simulink model "Automated_features1"  (R2020b)
settings: Solver=VariableStepAuto  StartTime=0.0  StopTime=10.0  RelTol=1e-3
undefined symbols (not defined in the file): sigbuilder_block
libraries: simulink x126
(part 2 of 3)

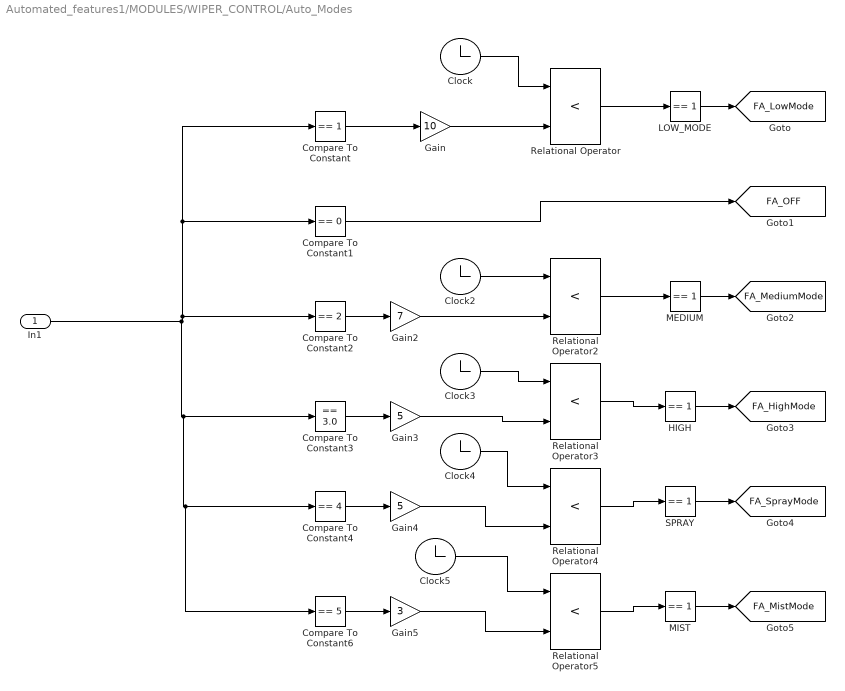
== system Automated_features1/MODULES/WIPER_CONTROL/Auto_Modes ==
  In1 : Inport
  Clock{,2..5} (5 alike) : Clock
      settings: Decimation=5
  Compare To Constant : simulink/Logic and Bit Operations/Compare To Constant  relop===  const=1  OutDataTypeStr=boolean
  Compare To Constant1 : simulink/Logic and Bit Operations/Compare To Constant  relop===  const=0  OutDataTypeStr=boolean
  Compare To Constant2 : simulink/Logic and Bit Operations/Compare To Constant  relop===  const=2  OutDataTypeStr=boolean
  Compare To Constant3 : simulink/Logic and Bit Operations/Compare To Constant  relop===  const=3.0  OutDataTypeStr=boolean
  Compare To Constant4 : simulink/Logic and Bit Operations/Compare To Constant  relop===  const=4  OutDataTypeStr=boolean
  Compare To Constant6 : simulink/Logic and Bit Operations/Compare To Constant  relop===  const=5  OutDataTypeStr=boolean
  Gain : Gain  Gain=10
  Gain2 : Gain  Gain=7
  Gain3 : Gain  Gain=5
  Gain4 : Gain  Gain=5
  Gain5 : Gain  Gain=3
  HIGH : simulink/Logic and Bit Operations/Compare To Constant  relop===  const=1  OutDataTypeStr=boolean
  LOW_MODE : simulink/Logic and Bit Operations/Compare To Constant  relop===  const=1  OutDataTypeStr=boolean
  MEDIUM : simulink/Logic and Bit Operations/Compare To Constant  relop===  const=1  OutDataTypeStr=boolean
  MIST : simulink/Logic and Bit Operations/Compare To Constant  relop===  const=1  OutDataTypeStr=boolean
  Relational Operator{,2..5} (5 alike) : RelationalOperator  Operator=<  OutDataTypeStr=boolean  RndMeth=Simplest
  SPRAY : simulink/Logic and Bit Operations/Compare To Constant  relop===  const=1  OutDataTypeStr=boolean
  tag scope: FA_HighMode=global, FA_LowMode=global, FA_MediumMode=global, FA_MistMode=global, FA_OFF=global, FA_SprayMode=global
  wires:
  In1/1 -> Compare To Constant6/1, Compare To Constant4/1, Compare To Constant3/1, Compare To Constant2/1, Compare To Constant/1, Compare To Constant1/1
  Clock/1 -> Relational Operator/1
  Relational Operator/1 -> LOW_MODE/1
  Gain/1 -> Relational Operator/2
  Compare To Constant/1 -> Gain/1
  Clock2/1 -> Relational Operator2/1
  Gain2/1 -> Relational Operator2/2
  Compare To Constant2/1 -> Gain2/1
  Clock3/1 -> Relational Operator3/1
  Gain3/1 -> Relational Operator3/2
  Compare To Constant3/1 -> Gain3/1
  Gain4/1 -> Relational Operator4/2
  Clock4/1 -> Relational Operator4/1
  Compare To Constant4/1 -> Gain4/1
  LOW_MODE/1 -> [FA_LowMode]
  MEDIUM/1 -> [FA_MediumMode]
  Relational Operator2/1 -> MEDIUM/1
  HIGH/1 -> [FA_HighMode]
  Relational Operator3/1 -> HIGH/1
  SPRAY/1 -> [FA_SprayMode]
  Relational Operator4/1 -> SPRAY/1
  Compare To Constant1/1 -> [FA_OFF]
  Relational Operator5/1 -> MIST/1
  Gain5/1 -> Relational Operator5/2
  Clock5/1 -> Relational Operator5/1
  MIST/1 -> [FA_MistMode]
  Compare To Constant6/1 -> Gain5/1

== system Automated_features1/MODULES/WIPER_CONTROL/Back_Windshield ==
  Lamp : LampBlock

== system Automated_features1/MODULES/WIPER_CONTROL/Front_Windshield ==
  Enable : EnablePort
  Auto_Modes : Subsystem
  Manual_mode : Subsystem
  Rotary Switch : RotarySwitchBlock  Commented=on
      settings: Values={{'Off', 'Low', 'Medium', 'High', 'Spray', 'Manual', 'MistMode'}, [0 1 2 3 4 5 6]}
  wires:
  [FW_Modes] -> Manual_mode/1(In1), Auto_Modes/1(In1)

== system Automated_features1/MODULES/WIPER_CONTROL/Manual_mode ==
  In1 : Inport
  Bw30_60 : Logic  IconShape=distinctive  AllPortsSameDT=off  OutDataTypeStr=boolean
  Bw60_100 : Logic  IconShape=distinctive  AllPortsSameDT=off  OutDataTypeStr=boolean
  Compare To Constant1 : simulink/Logic and Bit Operations/Compare To Constant  relop=>  const=30  OutDataTypeStr=boolean
  Compare To Constant2 : simulink/Logic and Bit Operations/Compare To Constant  relop=<=  const=60  OutDataTypeStr=boolean
  Compare To Constant3 : simulink/Logic and Bit Operations/Compare To Constant  relop=>  const=60  OutDataTypeStr=boolean
  Compare To Constant4 : simulink/Logic and Bit Operations/Compare To Constant  relop=<=  const=100  OutDataTypeStr=boolean
  Display : Display
  LessThan30 : simulink/Logic and Bit Operations/Compare To Constant  relop=<=  const=30  OutDataTypeStr=boolean
  Slider : SliderBlock
  String Constant : StringConstant  String="\"Undefined!\""
  Switch : Switch  Criteria=u2 > Threshold  Threshold=5
  tag scope: FM_Bw30_60=global, FM_Bw60_100=global, FM_lessthan30=global
  wires:
  Compare To Constant1/1 -> Bw30_60/1
  Bw30_60/1 -> [FM_Bw30_60]
  [FC_ManualInput] -> Compare To Constant4/1, Compare To Constant3/1, Compare To Constant2/1, Compare To Constant1/1, LessThan30/1, Switch/1
  Compare To Constant4/1 -> Bw60_100/2
  LessThan30/1 -> [FM_lessthan30]
  Switch/1 -> Display/1
  Compare To Constant3/1 -> Bw60_100/1
  Bw60_100/1 -> [FM_Bw60_100]
  Compare To Constant2/1 -> Bw30_60/2
  In1/1 -> Switch/2
  String Constant/1 -> Switch/3

== system Automated_features1/MODULES/WIPER_CONTROL/Wiper_Control ==
  Inport : Inport
  AND : Logic  IconShape=distinctive  AllPortsSameDT=off  OutDataTypeStr=boolean
  AND1 : Logic  IconShape=distinctive  AllPortsSameDT=off  OutDataTypeStr=boolean
  Atomic Subsystem : Subsystem  TreatAsAtomicUnit=on
  Atomic Subsystem1 : Subsystem  TreatAsAtomicUnit=on
  Back switch : SliderSwitchBlock  Commented=on
      settings: Values={{'Off', 'On'}, [0 1]}
  Back_Windshield : Subsystem  Commented=on  TreatAsAtomicUnit=on
  Front switch : SliderSwitchBlock  Commented=on
      settings: Values={{'Off', 'On'}, [0 1]}
  Front_Windshield : Subsystem  Commented=on  TreatAsAtomicUnit=on
  wires:
  Inport/1 -> AND1/2, AND/2
  [WC_FrontS] -> AND/1
  [WC_BackS] -> AND1/1
  AND1/1 -> Atomic Subsystem/1(Inport)
  AND/1 -> Atomic Subsystem1/1(Inport)

== system Automated_features1/MODULES/sunroof/Subsystem ==
  Enable : Inport
  Inport : Inport  Port=2
  Enabled Subsystem : Subsystem  TreatAsAtomicUnit=on
  Outport : Outport
  wires:
  Enabled Subsystem/1(Outport) -> Outport/1
  Inport/1 -> Enabled Subsystem/1(In1)
  Enable/1 -> Enabled Subsystem/Enable

== system Automated_features1/MODULES/sunroof/Subsystem1 ==
  Enable : Inport
  Inport : Inport  Port=2
  Enabled Subsystem1 : Subsystem  TreatAsAtomicUnit=on
  Outport : Outport
  wires:
  Inport/1 -> Enabled Subsystem1/1(In1)
  Enabled Subsystem1/1(Outport) -> Outport/1
  Enable/1 -> Enabled Subsystem1/Enable

== system Automated_features1/MODULES/sunroof/enabling system ==
  Chart : Stateflow chart  TreatAsAtomicUnit=on
      settings: PortSchema="{\"entries\":[{\"content\":{\"sides\":[{\"content\":{\"connectorIds\":[\"In2\",\"In1\"]},\"type\":\"ConnectorPlacement.EquallySpacedRectSide\",\"uuid\":\"e77fb548-5411-4dff-a09c-dcff2e4e83fa\"},{\"content\":{\"connectorIds\":[\"Out1\",\"Out2\"],\"side\":\"RIGHT\"},\"type\":\"ConnectorPlacement.EquallySpacedRectSide\",\"uuid\":\"fb2d12f5-730f-4265-a3f8-30409b75040e\"},{\"content\":{\"connectorIds\":[],\"side\":\"TOP\"},\"type\":\"ConnectorPlacement.EquallySpacedRectSide\",\"uuid\":\"5ec706c6-4a0b-4294-a183-09121d2d4adc\"},{\"content\":{\"connectorIds\":[],\"side\":\"HIDDEN\"},\"type\":\"ConnectorPlacement.EquallySpacedRectSide\",\"uuid\":\"e64ccab7-f9d3-41b0-81fa-c7461dca4746\"}]},\"type\":\"ConnectorPlacement.EquallySpacedConnector\",\"uuid\":\"e8c87857-404b-4a97-9417-fff31936aad1\"}],\"packageUris\":[\"http://schema.mathworks.com/mf0/Connector/R2020b\"],\"version\":\"1.0\"}"
  Outport : Outport
  enableO : Outport  Port=2
  wires:
  Chart/1(enableC) -> Outport/1
  [CL_SW] -> Chart/1(closeButton)
  Chart/2(enableO) -> enableO/1
  [OP_SW] -> Chart/2(openButton)

== system Automated_features1/MODULES/	POWER_WINDOW/Subsystem4/Front_left_subsystem ==
  lock/unlock : Inport
  In_fl_b : Inport  Port=2
  In_fl_Dc : Inport  Port=3
  object : Inport  Port=4
  Enable : EnablePort
  AND : Logic  IconShape=distinctive  AllPortsSameDT=off  OutDataTypeStr=boolean
  Compare To Constant1 : simulink/Logic and Bit Operations/Compare To Constant  relop===  const=1  OutDataTypeStr=boolean
  Display : Display
  Display1 : Display
  Scope : Scope  NumInputPorts=2
  Switch_lock_unlock : Switch  Criteria=u2 > Threshold
  check_ip : Constant
  decision_Box : Stateflow chart  TreatAsAtomicUnit=on
  inp_data : Logic  Operator=NXOR  IconShape=distinctive  AllPortsSameDT=off  OutDataTypeStr=boolean
  or1 : Logic  Operator=NXOR  IconShape=distinctive  AllPortsSameDT=off  OutDataTypeStr=boolean
  Outport : Outport
  Outport1 : Outport  Port=2
  tag scope: A=global
  wires:
  In_fl_b/1 -> AND/1
  check_ip/1 -> or1/1
  Switch_lock_unlock/1 -> [b1]
  Compare To Constant1/1 -> or1/2
  [b1] -> Display/1
  decision_Box/1(op1) -> Outport1/1, Switch_lock_unlock/3, Switch_lock_unlock/1, Scope/2, [A]
  decision_Box/2(warning) -> Outport/1, Scope/1
  object/1 -> decision_Box/2(data1)
  [A] -> Display1/1
  inp_data/1 -> decision_Box/1(data)
  In_fl_Dc/1 -> Compare To Constant1/1
  AND/1 -> inp_data/1  "res"
  or1/1 -> inp_data/2
  lock/unlock/1 -> Switch_lock_unlock/2, AND/2

== system Automated_features1/MODULES/	POWER_WINDOW/Subsystem4/Rear_right_Subsystem ==
  lock/unlock : Inport
  In2 : Inport  Port=2
  In3 : Inport  Port=3
  object : Inport  Port=4
  Enable : EnablePort
  Chart : Stateflow chart  TreatAsAtomicUnit=on
  Compare To Constant1 : simulink/Logic and Bit Operations/Compare To Constant  relop===  const=3  OutDataTypeStr=boolean
  Constant1 : Constant  Value=3
  Display2 : Display
  Display3 : Display
  Scope : Scope  NumInputPorts=2
  Switch : Switch  Criteria=u2 > Threshold
  or1 : Logic  Operator=NXOR  IconShape=distinctive  AllPortsSameDT=off  OutDataTypeStr=boolean
  or2 : Logic  IconShape=distinctive  AllPortsSameDT=off  OutDataTypeStr=boolean
  or3 : Logic  Operator=NXOR  IconShape=distinctive  AllPortsSameDT=off  OutDataTypeStr=boolean
  Outport : Outport
  Outport1 : Outport  Port=2
  tag scope: c=global
  wires:
  Constant1/1 -> or1/1
  [b3] -> Display2/1
  Compare To Constant1/1 -> or1/2
  Switch/1 -> [b3]
  lock/unlock/1 -> or2/2, Switch/2
  Chart/2(warning) -> Scope/1, Outport/1  "ss3"
  object/1 -> Chart/2(data1)
  or1/1 -> or3/2
  or2/1 -> or3/1  "res"
  or3/1 -> Chart/1(data)
  [c] -> Display3/1
  Chart/1(op1) -> Outport1/1, [c], Scope/2, Switch/3, Switch/1
  In2/1 -> or2/1
  In3/1 -> Compare To Constant1/1

== system Automated_features1/MODULES/	POWER_WINDOW/Subsystem4/driver_control_Subsystem ==
  In1 : Inport
  object : Inport  Port=2
  Enable : EnablePort
  Chart : Stateflow chart  TreatAsAtomicUnit=on
  Display4 : Display
  Scope : Scope  NumInputPorts=2
  Outport : Outport
  Outport1 : Outport  Port=2
  tag scope: d=global
  wires:
  Chart/2(warning) -> Outport/1, Scope/1  "ss4"
  object/1 -> Chart/2(data1)
  In1/1 -> Chart/1(data)
  [d] -> Display4/1
  Chart/1(op1) -> Outport1/1, [d], Scope/2

== system Automated_features1/MODULES/	POWER_WINDOW/Subsystem4/rear_left_Subsystem ==
  lock/unlock : Inport
  In2 : Inport  Port=2
  In3 : Inport  Port=3
  object : Inport  Port=4
  Enable : EnablePort
  Chart : Stateflow chart  TreatAsAtomicUnit=on
  Compare To Constant2 : simulink/Logic and Bit Operations/Compare To Constant  relop===  const=2  OutDataTypeStr=boolean
  Constant1 : Constant  Value=2
  Display1 : Display
  Display2 : Display
  Scope : Scope  NumInputPorts=2
  Switch1 : Switch  Criteria=u2 > Threshold
  or1 : Logic  Operator=NXOR  IconShape=distinctive  AllPortsSameDT=off  OutDataTypeStr=boolean
  or2 : Logic  Operator=NXOR  IconShape=distinctive  AllPortsSameDT=off  OutDataTypeStr=boolean
  or3 : Logic  IconShape=distinctive  AllPortsSameDT=off  OutDataTypeStr=boolean
  Outport : Outport
  Outport1 : Outport  Port=2
  tag scope: b=global
  wires:
  [b2] -> Display1/1
  Constant1/1 -> or2/1
  Compare To Constant2/1 -> or2/2
  Switch1/1 -> [b2]
  lock/unlock/1 -> Switch1/2, or3/2
  object/1 -> Chart/2(data1)
  Chart/2(warning) -> Outport/1, Scope/1  "ss2"
  or3/1 -> or1/1  "res"
  or2/1 -> or1/2
  or1/1 -> Chart/1(data)
  [b] -> Display2/1
  Chart/1(op1) -> Outport1/1, [b], Switch1/3, Switch1/1, Scope/2
  In2/1 -> or3/1
  In3/1 -> Compare To Constant2/1

== system Automated_features1/MODULES/Tire Pressure Monitoring System/TP_Monitoring/indicateHigh1 ==
  Enable : EnablePort
  Constant : Constant  Value=0
  Out1 : Outport
  wires:
  Constant/1 -> Out1/1

== system Automated_features1/MODULES/Tire Pressure Monitoring System/TP_Monitoring/indicateHigh2 ==
  Enable : EnablePort
  Constant : Constant  Value=0
  Out1 : Outport
  wires:
  Constant/1 -> Out1/1

== system Automated_features1/MODULES/Tire Pressure Monitoring System/TP_Monitoring/indicateHigh3 ==
  Enable : EnablePort
  Constant : Constant  Value=0
  Out1 : Outport
  wires:
  Constant/1 -> Out1/1

== system Automated_features1/MODULES/Tire Pressure Monitoring System/TP_Monitoring/indicateHigh4 ==
  Enable : EnablePort
  Constant : Constant  Value=0
  Out1 : Outport
  wires:
  Constant/1 -> Out1/1

== system Automated_features1/MODULES/Tire Pressure Monitoring System/TP_Monitoring/indicateLow1 ==
  Enable : EnablePort
  Constant : Constant
  Out1 : Outport
  wires:
  Constant/1 -> Out1/1

== system Automated_features1/MODULES/Tire Pressure Monitoring System/TP_Monitoring/indicateLow2 ==
  Enable : EnablePort
  Constant : Constant
  Out1 : Outport
  wires:
  Constant/1 -> Out1/1

== system Automated_features1/MODULES/Tire Pressure Monitoring System/TP_Monitoring/indicateLow3 ==
  Enable : EnablePort
  Constant : Constant
  Out1 : Outport
  wires:
  Constant/1 -> Out1/1

== system Automated_features1/MODULES/Tire Pressure Monitoring System/TP_Monitoring/indicateLow4 ==
  Enable : EnablePort
  Constant : Constant
  Out1 : Outport
  wires:
  Constant/1 -> Out1/1

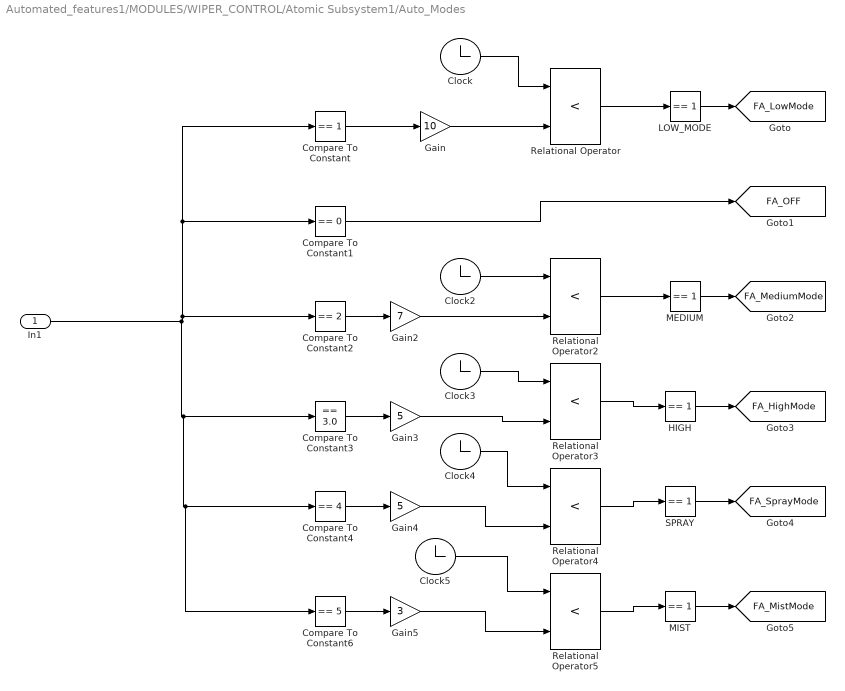
== system Automated_features1/MODULES/WIPER_CONTROL/Atomic Subsystem1/Auto_Modes ==
  In1 : Inport
  Clock{,2..5} (5 alike) : Clock
      settings: Decimation=5
  Compare To Constant : simulink/Logic and Bit Operations/Compare To Constant  relop===  const=1  OutDataTypeStr=boolean
  Compare To Constant1 : simulink/Logic and Bit Operations/Compare To Constant  relop===  const=0  OutDataTypeStr=boolean
  Compare To Constant2 : simulink/Logic and Bit Operations/Compare To Constant  relop===  const=2  OutDataTypeStr=boolean
  Compare To Constant3 : simulink/Logic and Bit Operations/Compare To Constant  relop===  const=3.0  OutDataTypeStr=boolean
  Compare To Constant4 : simulink/Logic and Bit Operations/Compare To Constant  relop===  const=4  OutDataTypeStr=boolean
  Compare To Constant6 : simulink/Logic and Bit Operations/Compare To Constant  relop===  const=5  OutDataTypeStr=boolean
  Gain : Gain  Gain=10
  Gain2 : Gain  Gain=7
  Gain3 : Gain  Gain=5
  Gain4 : Gain  Gain=5
  Gain5 : Gain  Gain=3
  HIGH : simulink/Logic and Bit Operations/Compare To Constant  relop===  const=1  OutDataTypeStr=boolean
  LOW_MODE : simulink/Logic and Bit Operations/Compare To Constant  relop===  const=1  OutDataTypeStr=boolean
  MEDIUM : simulink/Logic and Bit Operations/Compare To Constant  relop===  const=1  OutDataTypeStr=boolean
  MIST : simulink/Logic and Bit Operations/Compare To Constant  relop===  const=1  OutDataTypeStr=boolean
  Relational Operator{,2..5} (5 alike) : RelationalOperator  Operator=<  OutDataTypeStr=boolean  RndMeth=Simplest
  SPRAY : simulink/Logic and Bit Operations/Compare To Constant  relop===  const=1  OutDataTypeStr=boolean
  tag scope: FA_HighMode=global, FA_LowMode=global, FA_MediumMode=global, FA_MistMode=global, FA_OFF=global, FA_SprayMode=global
  wires:
  In1/1 -> Compare To Constant6/1, Compare To Constant4/1, Compare To Constant3/1, Compare To Constant2/1, Compare To Constant/1, Compare To Constant1/1
  Clock/1 -> Relational Operator/1
  Relational Operator/1 -> LOW_MODE/1
  Gain/1 -> Relational Operator/2
  Compare To Constant/1 -> Gain/1
  Clock2/1 -> Relational Operator2/1
  Gain2/1 -> Relational Operator2/2
  Compare To Constant2/1 -> Gain2/1
  Clock3/1 -> Relational Operator3/1
  Gain3/1 -> Relational Operator3/2
  Compare To Constant3/1 -> Gain3/1
  Gain4/1 -> Relational Operator4/2
  Clock4/1 -> Relational Operator4/1
  Compare To Constant4/1 -> Gain4/1
  LOW_MODE/1 -> [FA_LowMode]
  MEDIUM/1 -> [FA_MediumMode]
  Relational Operator2/1 -> MEDIUM/1
  HIGH/1 -> [FA_HighMode]
  Relational Operator3/1 -> HIGH/1
  SPRAY/1 -> [FA_SprayMode]
  Relational Operator4/1 -> SPRAY/1
  Compare To Constant1/1 -> [FA_OFF]
  Relational Operator5/1 -> MIST/1
  Gain5/1 -> Relational Operator5/2
  Clock5/1 -> Relational Operator5/1
  MIST/1 -> [FA_MistMode]
  Compare To Constant6/1 -> Gain5/1

== system Automated_features1/MODULES/WIPER_CONTROL/Atomic Subsystem1/Manual_mode ==
  In1 : Inport
  Bw30_60 : Logic  IconShape=distinctive  AllPortsSameDT=off  OutDataTypeStr=boolean
  Bw60_100 : Logic  IconShape=distinctive  AllPortsSameDT=off  OutDataTypeStr=boolean
  Compare To Constant1 : simulink/Logic and Bit Operations/Compare To Constant  relop=>  const=30  OutDataTypeStr=boolean
  Compare To Constant2 : simulink/Logic and Bit Operations/Compare To Constant  relop=<=  const=60  OutDataTypeStr=boolean
  Compare To Constant3 : simulink/Logic and Bit Operations/Compare To Constant  relop=>  const=60  OutDataTypeStr=boolean
  Compare To Constant4 : simulink/Logic and Bit Operations/Compare To Constant  relop=<=  const=100  OutDataTypeStr=boolean
  Display : Display
  LessThan30 : simulink/Logic and Bit Operations/Compare To Constant  relop=<=  const=30  OutDataTypeStr=boolean
  Slider : SliderBlock
  String Constant : StringConstant  String="\"Undefined!\""
  Switch : Switch  Criteria=u2 > Threshold  Threshold=5
  tag scope: FM_Bw30_60=global, FM_Bw60_100=global, FM_lessthan30=global
  wires:
  Compare To Constant1/1 -> Bw30_60/1
  Bw30_60/1 -> [FM_Bw30_60]
  [FC_ManualInput] -> Compare To Constant4/1, Compare To Constant3/1, Compare To Constant2/1, Compare To Constant1/1, LessThan30/1, Switch/1
  Compare To Constant4/1 -> Bw60_100/2
  LessThan30/1 -> [FM_lessthan30]
  Switch/1 -> Display/1
  Compare To Constant3/1 -> Bw60_100/1
  Bw60_100/1 -> [FM_Bw60_100]
  Compare To Constant2/1 -> Bw30_60/2
  In1/1 -> Switch/2
  String Constant/1 -> Switch/3

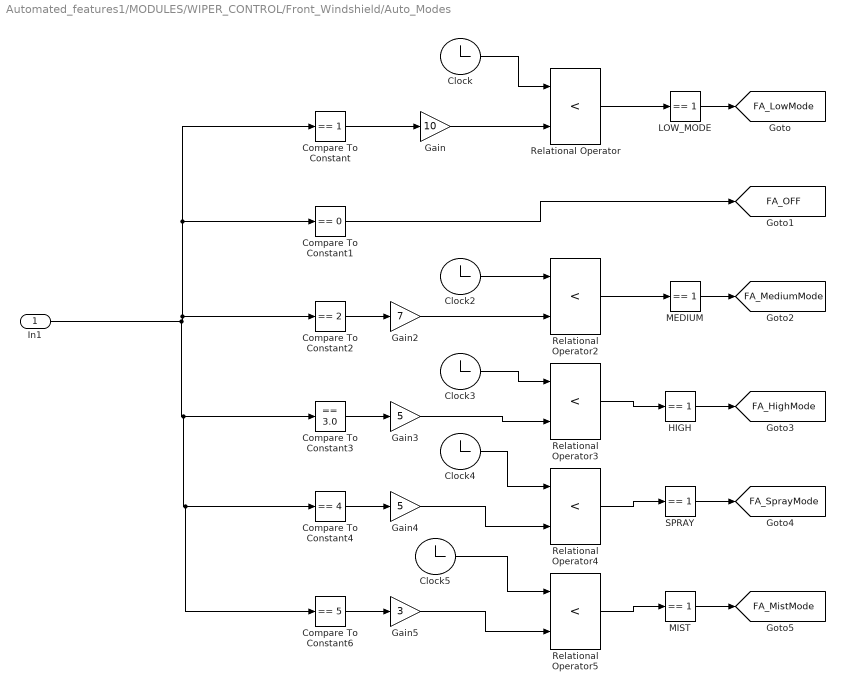
== system Automated_features1/MODULES/WIPER_CONTROL/Front_Windshield/Auto_Modes ==
  In1 : Inport
  Clock{,2..5} (5 alike) : Clock
      settings: Decimation=5
  Compare To Constant : simulink/Logic and Bit Operations/Compare To Constant  relop===  const=1  OutDataTypeStr=boolean
  Compare To Constant1 : simulink/Logic and Bit Operations/Compare To Constant  relop===  const=0  OutDataTypeStr=boolean
  Compare To Constant2 : simulink/Logic and Bit Operations/Compare To Constant  relop===  const=2  OutDataTypeStr=boolean
  Compare To Constant3 : simulink/Logic and Bit Operations/Compare To Constant  relop===  const=3.0  OutDataTypeStr=boolean
  Compare To Constant4 : simulink/Logic and Bit Operations/Compare To Constant  relop===  const=4  OutDataTypeStr=boolean
  Compare To Constant6 : simulink/Logic and Bit Operations/Compare To Constant  relop===  const=5  OutDataTypeStr=boolean
  Gain : Gain  Gain=10
  Gain2 : Gain  Gain=7
  Gain3 : Gain  Gain=5
  Gain4 : Gain  Gain=5
  Gain5 : Gain  Gain=3
  HIGH : simulink/Logic and Bit Operations/Compare To Constant  relop===  const=1  OutDataTypeStr=boolean
  LOW_MODE : simulink/Logic and Bit Operations/Compare To Constant  relop===  const=1  OutDataTypeStr=boolean
  MEDIUM : simulink/Logic and Bit Operations/Compare To Constant  relop===  const=1  OutDataTypeStr=boolean
  MIST : simulink/Logic and Bit Operations/Compare To Constant  relop===  const=1  OutDataTypeStr=boolean
  Relational Operator{,2..5} (5 alike) : RelationalOperator  Operator=<  OutDataTypeStr=boolean  RndMeth=Simplest
  SPRAY : simulink/Logic and Bit Operations/Compare To Constant  relop===  const=1  OutDataTypeStr=boolean
  tag scope: FA_HighMode=global, FA_LowMode=global, FA_MediumMode=global, FA_MistMode=global, FA_OFF=global, FA_SprayMode=global
  wires:
  In1/1 -> Compare To Constant6/1, Compare To Constant4/1, Compare To Constant3/1, Compare To Constant2/1, Compare To Constant/1, Compare To Constant1/1
  Clock/1 -> Relational Operator/1
  Relational Operator/1 -> LOW_MODE/1
  Gain/1 -> Relational Operator/2
  Compare To Constant/1 -> Gain/1
  Clock2/1 -> Relational Operator2/1
  Gain2/1 -> Relational Operator2/2
  Compare To Constant2/1 -> Gain2/1
  Clock3/1 -> Relational Operator3/1
  Gain3/1 -> Relational Operator3/2
  Compare To Constant3/1 -> Gain3/1
  Gain4/1 -> Relational Operator4/2
  Clock4/1 -> Relational Operator4/1
  Compare To Constant4/1 -> Gain4/1
  LOW_MODE/1 -> [FA_LowMode]
  MEDIUM/1 -> [FA_MediumMode]
  Relational Operator2/1 -> MEDIUM/1
  HIGH/1 -> [FA_HighMode]
  Relational Operator3/1 -> HIGH/1
  SPRAY/1 -> [FA_SprayMode]
  Relational Operator4/1 -> SPRAY/1
  Compare To Constant1/1 -> [FA_OFF]
  Relational Operator5/1 -> MIST/1
  Gain5/1 -> Relational Operator5/2
  Clock5/1 -> Relational Operator5/1
  MIST/1 -> [FA_MistMode]
  Compare To Constant6/1 -> Gain5/1

== system Automated_features1/MODULES/WIPER_CONTROL/Front_Windshield/Manual_mode ==
  In1 : Inport
  Bw30_60 : Logic  IconShape=distinctive  AllPortsSameDT=off  OutDataTypeStr=boolean
  Bw60_100 : Logic  IconShape=distinctive  AllPortsSameDT=off  OutDataTypeStr=boolean
  Compare To Constant1 : simulink/Logic and Bit Operations/Compare To Constant  relop=>  const=30  OutDataTypeStr=boolean
  Compare To Constant2 : simulink/Logic and Bit Operations/Compare To Constant  relop=<=  const=60  OutDataTypeStr=boolean
  Compare To Constant3 : simulink/Logic and Bit Operations/Compare To Constant  relop=>  const=60  OutDataTypeStr=boolean
  Compare To Constant4 : simulink/Logic and Bit Operations/Compare To Constant  relop=<=  const=100  OutDataTypeStr=boolean
  Display : Display
  LessThan30 : simulink/Logic and Bit Operations/Compare To Constant  relop=<=  const=30  OutDataTypeStr=boolean
  Slider : SliderBlock
  String Constant : StringConstant  String="\"Undefined!\""
  Switch : Switch  Criteria=u2 > Threshold  Threshold=5
  tag scope: FM_Bw30_60=global, FM_Bw60_100=global, FM_lessthan30=global
  wires:
  Compare To Constant1/1 -> Bw30_60/1
  Bw30_60/1 -> [FM_Bw30_60]
  [FC_ManualInput] -> Compare To Constant4/1, Compare To Constant3/1, Compare To Constant2/1, Compare To Constant1/1, LessThan30/1, Switch/1
  Compare To Constant4/1 -> Bw60_100/2
  LessThan30/1 -> [FM_lessthan30]
  Switch/1 -> Display/1
  Compare To Constant3/1 -> Bw60_100/1
  Bw60_100/1 -> [FM_Bw60_100]
  Compare To Constant2/1 -> Bw30_60/2
  In1/1 -> Switch/2
  String Constant/1 -> Switch/3

== system Automated_features1/MODULES/WIPER_CONTROL/Wiper_Control/Atomic Subsystem ==
  Inport : Inport
  Clock : Clock
      settings: Decimation=5
  Compare To Constant : simulink/Logic and Bit Operations/Compare To Constant  relop===  const=1  OutDataTypeStr=boolean
  Compare To Constant5 : simulink/Logic and Bit Operations/Compare To Constant  relop===  const=1  OutDataTypeStr=boolean
  Gain : Gain  Gain=10
  Relational Operator : RelationalOperator  Operator=<  OutDataTypeStr=boolean  RndMeth=Simplest
  tag scope: BW_Display=global
  wires:
  Compare To Constant5/1 -> [BW_Display]
  Inport/1 -> Compare To Constant/1
  Gain/1 -> Relational Operator/2
  Clock/1 -> Relational Operator/1
  Relational Operator/1 -> Compare To Constant5/1
  Compare To Constant/1 -> Gain/1

== system Automated_features1/MODULES/WIPER_CONTROL/Wiper_Control/Atomic Subsystem1 ==
  Inport : Inport
  Auto_Modes : Subsystem
  Display : Display
  Manual_mode : Subsystem
  wires:
  [FW_Modes] -> Manual_mode/1(In1), Auto_Modes/1(In1)
  Inport/1 -> Display/1

== system Automated_features1/MODULES/WIPER_CONTROL/Wiper_Control/Back_Windshield ==
  Lamp : LampBlock

== system Automated_features1/MODULES/WIPER_CONTROL/Wiper_Control/Front_Windshield ==
  Enable : EnablePort
  Auto_Modes : Subsystem
  Manual_mode : Subsystem
  Rotary Switch : RotarySwitchBlock  Commented=on
      settings: Values={{'Off', 'Low', 'Medium', 'High', 'Spray', 'Manual', 'MistMode'}, [0 1 2 3 4 5 6]}
  wires:
  [FW_Modes] -> Manual_mode/1(In1), Auto_Modes/1(In1)

== system Automated_features1/MODULES/sunroof/Subsystem/Enabled Subsystem ==
  In1 : Inport
  Enable : EnablePort
  Outport : Outport
  wires:
  In1/1 -> Outport/1

== system Automated_features1/MODULES/sunroof/Subsystem1/Enabled Subsystem1 ==
  In1 : Inport
  Enable : EnablePort
  Outport : Outport
  wires:
  In1/1 -> Outport/1

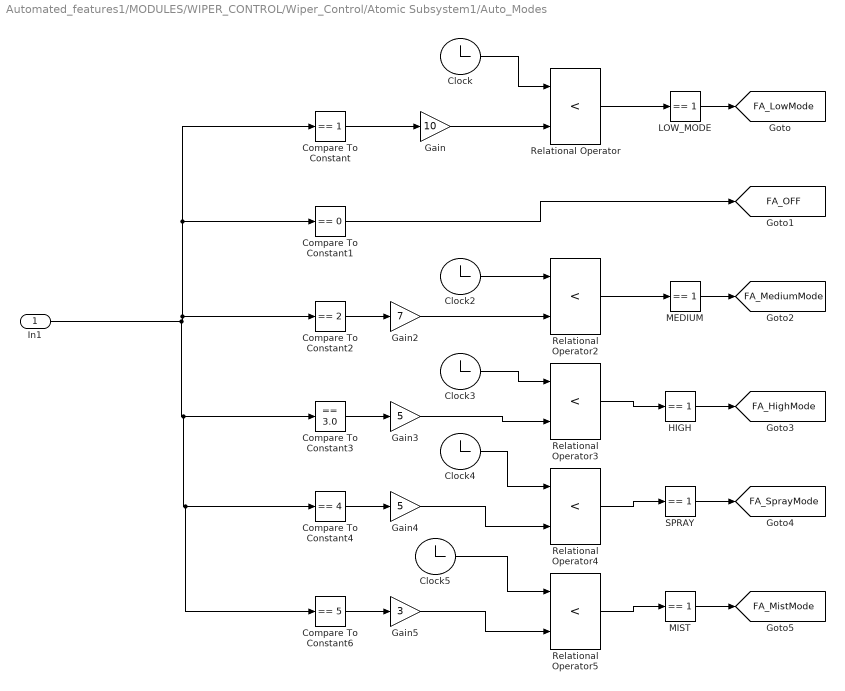
== system Automated_features1/MODULES/WIPER_CONTROL/Wiper_Control/Atomic Subsystem1/Auto_Modes ==
  In1 : Inport
  Clock{,2..5} (5 alike) : Clock
      settings: Decimation=5
  Compare To Constant : simulink/Logic and Bit Operations/Compare To Constant  relop===  const=1  OutDataTypeStr=boolean
  Compare To Constant1 : simulink/Logic and Bit Operations/Compare To Constant  relop===  const=0  OutDataTypeStr=boolean
  Compare To Constant2 : simulink/Logic and Bit Operations/Compare To Constant  relop===  const=2  OutDataTypeStr=boolean
  Compare To Constant3 : simulink/Logic and Bit Operations/Compare To Constant  relop===  const=3.0  OutDataTypeStr=boolean
  Compare To Constant4 : simulink/Logic and Bit Operations/Compare To Constant  relop===  const=4  OutDataTypeStr=boolean
  Compare To Constant6 : simulink/Logic and Bit Operations/Compare To Constant  relop===  const=5  OutDataTypeStr=boolean
  Gain : Gain  Gain=10
  Gain2 : Gain  Gain=7
  Gain3 : Gain  Gain=5
  Gain4 : Gain  Gain=5
  Gain5 : Gain  Gain=3
  HIGH : simulink/Logic and Bit Operations/Compare To Constant  relop===  const=1  OutDataTypeStr=boolean
  LOW_MODE : simulink/Logic and Bit Operations/Compare To Constant  relop===  const=1  OutDataTypeStr=boolean
  MEDIUM : simulink/Logic and Bit Operations/Compare To Constant  relop===  const=1  OutDataTypeStr=boolean
  MIST : simulink/Logic and Bit Operations/Compare To Constant  relop===  const=1  OutDataTypeStr=boolean
  Relational Operator{,2..5} (5 alike) : RelationalOperator  Operator=<  OutDataTypeStr=boolean  RndMeth=Simplest
  SPRAY : simulink/Logic and Bit Operations/Compare To Constant  relop===  const=1  OutDataTypeStr=boolean
  tag scope: FA_HighMode=global, FA_LowMode=global, FA_MediumMode=global, FA_MistMode=global, FA_OFF=global, FA_SprayMode=global
  wires:
  In1/1 -> Compare To Constant6/1, Compare To Constant4/1, Compare To Constant3/1, Compare To Constant2/1, Compare To Constant/1, Compare To Constant1/1
  Clock/1 -> Relational Operator/1
  Relational Operator/1 -> LOW_MODE/1
  Gain/1 -> Relational Operator/2
  Compare To Constant/1 -> Gain/1
  Clock2/1 -> Relational Operator2/1
  Gain2/1 -> Relational Operator2/2
  Compare To Constant2/1 -> Gain2/1
  Clock3/1 -> Relational Operator3/1
  Gain3/1 -> Relational Operator3/2
  Compare To Constant3/1 -> Gain3/1
  Gain4/1 -> Relational Operator4/2
  Clock4/1 -> Relational Operator4/1
  Compare To Constant4/1 -> Gain4/1
  LOW_MODE/1 -> [FA_LowMode]
  MEDIUM/1 -> [FA_MediumMode]
  Relational Operator2/1 -> MEDIUM/1
  HIGH/1 -> [FA_HighMode]
  Relational Operator3/1 -> HIGH/1
  SPRAY/1 -> [FA_SprayMode]
  Relational Operator4/1 -> SPRAY/1
  Compare To Constant1/1 -> [FA_OFF]
  Relational Operator5/1 -> MIST/1
  Gain5/1 -> Relational Operator5/2
  Clock5/1 -> Relational Operator5/1
  MIST/1 -> [FA_MistMode]
  Compare To Constant6/1 -> Gain5/1

== system Automated_features1/MODULES/WIPER_CONTROL/Wiper_Control/Atomic Subsystem1/Manual_mode ==
  In1 : Inport
  Bw30_60 : Logic  IconShape=distinctive  AllPortsSameDT=off  OutDataTypeStr=boolean
  Bw60_100 : Logic  IconShape=distinctive  AllPortsSameDT=off  OutDataTypeStr=boolean
  Compare To Constant1 : simulink/Logic and Bit Operations/Compare To Constant  relop=>  const=30  OutDataTypeStr=boolean
  Compare To Constant2 : simulink/Logic and Bit Operations/Compare To Constant  relop=<=  const=60  OutDataTypeStr=boolean
  Compare To Constant3 : simulink/Logic and Bit Operations/Compare To Constant  relop=>  const=60  OutDataTypeStr=boolean
  Compare To Constant4 : simulink/Logic and Bit Operations/Compare To Constant  relop=<=  const=100  OutDataTypeStr=boolean
  Display : Display
  LessThan30 : simulink/Logic and Bit Operations/Compare To Constant  relop=<=  const=30  OutDataTypeStr=boolean
  Slider : SliderBlock
  String Constant : StringConstant  String="\"Undefined!\""
  Switch : Switch  Criteria=u2 > Threshold  Threshold=5
  tag scope: FM_Bw30_60=global, FM_Bw60_100=global, FM_lessthan30=global
  wires:
  Compare To Constant1/1 -> Bw30_60/1
  Bw30_60/1 -> [FM_Bw30_60]
  [FC_ManualInput] -> Compare To Constant4/1, Compare To Constant3/1, Compare To Constant2/1, Compare To Constant1/1, LessThan30/1, Switch/1
  Compare To Constant4/1 -> Bw60_100/2
  LessThan30/1 -> [FM_lessthan30]
  Switch/1 -> Display/1
  Compare To Constant3/1 -> Bw60_100/1
  Bw60_100/1 -> [FM_Bw60_100]
  Compare To Constant2/1 -> Bw30_60/2
  In1/1 -> Switch/2
  String Constant/1 -> Switch/3

== system Automated_features1/MODULES/WIPER_CONTROL/Wiper_Control/Front_Windshield/Auto_Modes ==
  In1 : Inport
  Clock{,2..5} (5 alike) : Clock
      settings: Decimation=5
  Compare To Constant : simulink/Logic and Bit Operations/Compare To Constant  relop===  const=1  OutDataTypeStr=boolean
  Compare To Constant1 : simulink/Logic and Bit Operations/Compare To Constant  relop===  const=0  OutDataTypeStr=boolean
  Compare To Constant2 : simulink/Logic and Bit Operations/Compare To Constant  relop===  const=2  OutDataTypeStr=boolean
  Compare To Constant3 : simulink/Logic and Bit Operations/Compare To Constant  relop===  const=3.0  OutDataTypeStr=boolean
  Compare To Constant4 : simulink/Logic and Bit Operations/Compare To Constant  relop===  const=4  OutDataTypeStr=boolean
  Compare To Constant6 : simulink/Logic and Bit Operations/Compare To Constant  relop===  const=5  OutDataTypeStr=boolean
  Gain : Gain  Gain=10
  Gain2 : Gain  Gain=7
  Gain3 : Gain  Gain=5
  Gain4 : Gain  Gain=5
  Gain5 : Gain  Gain=3
  HIGH : simulink/Logic and Bit Operations/Compare To Constant  relop===  const=1  OutDataTypeStr=boolean
  LOW_MODE : simulink/Logic and Bit Operations/Compare To Constant  relop===  const=1  OutDataTypeStr=boolean
  MEDIUM : simulink/Logic and Bit Operations/Compare To Constant  relop===  const=1  OutDataTypeStr=boolean
  MIST : simulink/Logic and Bit Operations/Compare To Constant  relop===  const=1  OutDataTypeStr=boolean
  Relational Operator{,2..5} (5 alike) : RelationalOperator  Operator=<  OutDataTypeStr=boolean  RndMeth=Simplest
  SPRAY : simulink/Logic and Bit Operations/Compare To Constant  relop===  const=1  OutDataTypeStr=boolean
  tag scope: FA_HighMode=global, FA_LowMode=global, FA_MediumMode=global, FA_MistMode=global, FA_OFF=global, FA_SprayMode=global
  wires:
  In1/1 -> Compare To Constant6/1, Compare To Constant4/1, Compare To Constant3/1, Compare To Constant2/1, Compare To Constant/1, Compare To Constant1/1
  Clock/1 -> Relational Operator/1
  Relational Operator/1 -> LOW_MODE/1
  Gain/1 -> Relational Operator/2
  Compare To Constant/1 -> Gain/1
  Clock2/1 -> Relational Operator2/1
  Gain2/1 -> Relational Operator2/2
  Compare To Constant2/1 -> Gain2/1
  Clock3/1 -> Relational Operator3/1
  Gain3/1 -> Relational Operator3/2
  Compare To Constant3/1 -> Gain3/1
  Gain4/1 -> Relational Operator4/2
  Clock4/1 -> Relational Operator4/1
  Compare To Constant4/1 -> Gain4/1
  LOW_MODE/1 -> [FA_LowMode]
  MEDIUM/1 -> [FA_MediumMode]
  Relational Operator2/1 -> MEDIUM/1
  HIGH/1 -> [FA_HighMode]
  Relational Operator3/1 -> HIGH/1
  SPRAY/1 -> [FA_SprayMode]
  Relational Operator4/1 -> SPRAY/1
  Compare To Constant1/1 -> [FA_OFF]
  Relational Operator5/1 -> MIST/1
  Gain5/1 -> Relational Operator5/2
  Clock5/1 -> Relational Operator5/1
  MIST/1 -> [FA_MistMode]
  Compare To Constant6/1 -> Gain5/1

== system Automated_features1/MODULES/WIPER_CONTROL/Wiper_Control/Front_Windshield/Manual_mode ==
  In1 : Inport
  Bw30_60 : Logic  IconShape=distinctive  AllPortsSameDT=off  OutDataTypeStr=boolean
  Bw60_100 : Logic  IconShape=distinctive  AllPortsSameDT=off  OutDataTypeStr=boolean
  Compare To Constant1 : simulink/Logic and Bit Operations/Compare To Constant  relop=>  const=30  OutDataTypeStr=boolean
  Compare To Constant2 : simulink/Logic and Bit Operations/Compare To Constant  relop=<=  const=60  OutDataTypeStr=boolean
  Compare To Constant3 : simulink/Logic and Bit Operations/Compare To Constant  relop=>  const=60  OutDataTypeStr=boolean
  Compare To Constant4 : simulink/Logic and Bit Operations/Compare To Constant  relop=<=  const=100  OutDataTypeStr=boolean
  Display : Display
  LessThan30 : simulink/Logic and Bit Operations/Compare To Constant  relop=<=  const=30  OutDataTypeStr=boolean
  Slider : SliderBlock
  String Constant : StringConstant  String="\"Undefined!\""
  Switch : Switch  Criteria=u2 > Threshold  Threshold=5
  tag scope: FM_Bw30_60=global, FM_Bw60_100=global, FM_lessthan30=global
  wires:
  Compare To Constant1/1 -> Bw30_60/1
  Bw30_60/1 -> [FM_Bw30_60]
  [FC_ManualInput] -> Compare To Constant4/1, Compare To Constant3/1, Compare To Constant2/1, Compare To Constant1/1, LessThan30/1, Switch/1
  Compare To Constant4/1 -> Bw60_100/2
  LessThan30/1 -> [FM_lessthan30]
  Switch/1 -> Display/1
  Compare To Constant3/1 -> Bw60_100/1
  Bw60_100/1 -> [FM_Bw60_100]
  Compare To Constant2/1 -> Bw30_60/2
  In1/1 -> Switch/2
  String Constant/1 -> Switch/3

== stateflow chart Automated_features1/MODULES/sunroof/enabling system/Chart ==
  state stage1
    entry:
    enableO=0;
    enableC=0;
  state stage3
    entry:
    enableO=1;
    enableC=0;
  state stage2
    entry:
    enableO=0;
    enableC=1;
  (default) -> stage1
  stage1 -> stage3 [order 3] : [openButton ==1 && closeButton==0]
  stage1 -> stage2 [order 1] : [openButton ==0 && closeButton==1]
  stage2 -> stage1 : [(openButton ==1 && closeButton==1) || (openButton ==0 && closeButton==0)]
  stage3 -> stage1 : [(openButton ==1 && closeButton==1) || (openButton ==0 && closeButton==0)]
  stage1 -> stage1 [order 2] : [(openButton ==1 && closeButton==1) || (openButton ==0 && closeButton==0)]
  data: closeButton input; openButton input; enableC output; enableO output

== matlab function Automated_features1/MODULES/AIRBAGSYSTEM/ActivateAirBagSensor ==
  data: SuddenDeceleration input; AirBagSensor output
function AirBagSensor  = fcn(SuddenDeceleration)
if SuddenDeceleration == 1
         %Front airbag active
   AirBagSensor = 1;
else 
   AirBagSensor = 0;   
end

== matlab function Automated_features1/MODULES/AIRBAGSYSTEM/FrontAirBagActivation/WeightSensor ==
  data: driver input; DRIVER output; l_front input; L_FRONT output; l_rear input; r_rear input; L_REAR output; R_REAR output
function [DRIVER,L_FRONT,L_REAR,R_REAR] = fcn(driver, l_front,l_rear,r_rear)
    if (driver==0 && l_front==0 && l_rear==0 && r_rear==1)      %0001
        DRIVER=0;
        L_FRONT=0;
        L_REAR=0;
        R_REAR=1;
    
    elseif (driver==0 && l_front==0 && l_rear==1 && r_rear==0)
        DRIVER=0;
        L_FRONT=0;
        L_REAR=1;
        R_REAR=0;
    
    elseif (driver==0 && l_front==0 && l_rear==1 && r_rear==1)
        DRIVER=0;
        L_FRONT=0;
        L_REAR=1;
        R_REAR=1;

    elseif (driver==0 && l_front==1 && l_rear==0 && r_rear==0)
        DRIVER=0;
        L_FRONT=1;
        L_REAR=0;
        R_REAR=0;
    
    elseif (driver==0 && l_front==1 && l_rear==0 && r_rear==1)
        DRIVER=0;
        L_FRONT=1;
        L_REAR=0;
        R_REAR=1;
    
    elseif (driver==0 && l_front==1 && l_rear==1 && r_rear==0)
        DRIVER=0;
        L_FRONT=1;
        L_REAR=1;
        R_REAR=0;
    
    elseif (driver==0 && l_front==1 && l_rear==1 && r_rear==1)
        DRIVER=0;
        L_FRONT=1;
        L_REAR=1;
        R_REAR=1;
    
    elseif (driver==1 && l_front==0 && l_rear==0 && r_rear==0)
        DRIVER=1;
        L_FRONT=0;
        L_REAR=0;
        R_REAR=0;
    
    elseif (driver==1 && l_front==0 && l_rear==0 && r_rear==1)
        DRIVER=1;
        L_FRONT=0;
        L_REAR=0;
        R_REAR=1;
    
    elseif (driver==1 && l_front==0 && l_rear==1 && r_rear==0)
        DRIVER=1;
        L_FRONT=0;
        L_REAR=1;
        R_REAR=0;
    
    elseif (driver==1 && l_front==0 && l_rear==1 && r_rear==1)
        DRIVER=1;
        L_FRONT=0;
        L_REAR=1;
        R_REAR=1;
    
    elseif (driver==1 && l_front==1 && l_rear==0 && r_rear==0)
        DRIVER=1;
        L_FRONT=1;
        L_REAR=0;
        R_REAR=0;
    
    elseif (driver==1 && l_front==1 && l_rear==0 && r_rear==1)
        DRIVER=1;
        L_FRONT=1;
        L_REAR=0;
        R_REAR=1;
    
    elseif (driver==1 && l_front==1 && l_rear==1 && r_rear==0)
        DRIVER=1;
        L_FRONT=1;
        L_REAR=1;
        R_REAR=0;
    
    elseif (driver==1 && l_front==1 && l_rear==1 && r_rear==1)
        DRIVER=1;
        L_FRONT=1;
        L_REAR=1;
        R_REAR=1;
    
    else
        DRIVER=0;
        L_FRONT=0;
        L_REAR=0;
        R_REAR=0;
    end

== matlab function Automated_features1/MODULES/AIRBAGSYSTEM/SideAirBagActivation1/WeightSensor ==
  data: driver input; DRIVER output; l_front input; L_FRONT output; l_rear input; r_rear input; L_REAR output; R_REAR output
function [DRIVER,L_FRONT,L_REAR,R_REAR] = fcn(driver, l_front,l_rear,r_rear)
    if (driver==0 && l_front==0 && l_rear==0 && r_rear==1)      %0001
        DRIVER=0;
        L_FRONT=0;
        L_REAR=0;
        R_REAR=1;
    
    elseif (driver==0 && l_front==0 && l_rear==1 && r_rear==0)
        DRIVER=0;
        L_FRONT=0;
        L_REAR=1;
        R_REAR=0;
    
    elseif (driver==0 && l_front==0 && l_rear==1 && r_rear==1)
        DRIVER=0;
        L_FRONT=0;
        L_REAR=1;
        R_REAR=1;

    elseif (driver==0 && l_front==1 && l_rear==0 && r_rear==0)
        DRIVER=0;
        L_FRONT=1;
        L_REAR=0;
        R_REAR=0;
    
    elseif (driver==0 && l_front==1 && l_rear==0 && r_rear==1)
        DRIVER=0;
        L_FRONT=1;
        L_REAR=0;
        R_REAR=1;
    
    elseif (driver==0 && l_front==1 && l_rear==1 && r_rear==0)
        DRIVER=0;
        L_FRONT=1;
        L_REAR=1;
        R_REAR=0;
    
    elseif (driver==0 && l_front==1 && l_rear==1 && r_rear==1)
        DRIVER=0;
        L_FRONT=1;
        L_REAR=1;
        R_REAR=1;
    
    elseif (driver==1 && l_front==0 && l_rear==0 && r_rear==0)
        DRIVER=1;
        L_FRONT=0;
        L_REAR=0;
        R_REAR=0;
    
    elseif (driver==1 && l_front==0 && l_rear==0 && r_rear==1)
        DRIVER=1;
        L_FRONT=0;
        L_REAR=0;
        R_REAR=1;
    
    elseif (driver==1 && l_front==0 && l_rear==1 && r_rear==0)
        DRIVER=1;
        L_FRONT=0;
        L_REAR=1;
        R_REAR=0;
    
    elseif (driver==1 && l_front==0 && l_rear==1 && r_rear==1)
        DRIVER=1;
        L_FRONT=0;
        L_REAR=1;
        R_REAR=1;
    
    elseif (driver==1 && l_front==1 && l_rear==0 && r_rear==0)
        DRIVER=1;
        L_FRONT=1;
        L_REAR=0;
        R_REAR=0;
    
    elseif (driver==1 && l_front==1 && l_rear==0 && r_rear==1)
        DRIVER=1;
        L_FRONT=1;
        L_REAR=0;
        R_REAR=1;
    
    elseif (driver==1 && l_front==1 && l_rear==1 && r_rear==0)
        DRIVER=1;
        L_FRONT=1;
        L_REAR=1;
        R_REAR=0;
    
    elseif (driver==1 && l_front==1 && l_rear==1 && r_rear==1)
        DRIVER=1;
        L_FRONT=1;
        L_REAR=1;
        R_REAR=1;
    
    else
        DRIVER=0;
        L_FRONT=0;
        L_REAR=0;
        R_REAR=0;
    end

== matlab function Automated_features1/MODULES/CRUISE_CONTROL/MATLAB Function ==
  data: ESC_CC input; TSC_CC input; BRAKE_CC input; IGN input; y output; DESIRED_SPEED_CRUISE input; cs input; CRUISE_SPEED_CHANGE_SW input; speedch input
function y = fcn(ESC_CC, TSC_CC, BRAKE_CC, IGN, DESIRED_SPEED_CRUISE, cs, CRUISE_SPEED_CHANGE_SW, speedch)

if (IGN==1&& ESC_CC==0 &&TSC_CC==0 && BRAKE_CC==0)
    if (cs ==1 && DESIRED_SPEED_CRUISE>40 && CRUISE_SPEED_CHANGE_SW==1)
        y= DESIRED_SPEED_CRUISE+speedch;
    else
        y=DESIRED_SPEED_CRUISE;
    end
      
else
    y=0;
end

== stateflow chart Automated_features1/MODULES/	POWER_WINDOW/Subsystem4/Front_left_subsystem/decision_Box ==
  state Normal
    state Start
      entry:
      op1 = 25;
    state second
      entry:
      op1 = 100;
    state PrepareToStop
      entry:
      op1 = 75;
    state Go
      % Green light
      entry:
      op1 = 50;
    (default) -> Start
    Start -> (junction 9)
    (junction 9) -> (junction 6) : after(1,sec)
    PrepareToStop -> second : after(1,sec)
    (junction 6) -> Go
    Go -> PrepareToStop : after(1,sec)
  state Fault
    entry:
    op1 =0;
    state BlinkOn
      % Red light
      entry:
      warning = 1;
    (default) -> BlinkOn
  state block_start
    entry:
  state Normal2
    state state5
      entry:
      op1=0
    state Start1
      entry:
      op1=op1;
    state two
      entry:
      op1 = 0;
    state four3
      entry:
      op1 = 0;
    state three
      entry:
      op1 = 25;
    state three1
      entry:
      op1 = 0;
    state five2
      entry:
      op1=0;
    state five
      entry:
      op1=50;
    state five1
      entry:
      op1=25;
    state four2
      entry:
      op1 = 25;
    state four
      entry:
      op1 = 75;
    state four1
      entry:
      op1 = 50;
    Start1 -> state5 [order 4] : [op1==0]
    (default) -> Start1
    Start1 -> (junction 143) [order 2] : after(1,sec)[op1==25]
    (junction 143) -> four3
    Start1 -> (junction 89) [order 3]
    Start1 -> (junction 103) [order 5]
    Start1 -> (junction 48) [order 1]
    (junction 103) -> (junction 104) : after(1,sec)[op1==50]
    (junction 48) -> (junction 49) : after(1,sec)[op1==100]
    (junction 89) -> (junction 90) : after(1,sec)[op1==75]
    three -> two : after(1,sec)[op1==25]
    (junction 104) -> four2
    (junction 49) -> four
    five -> three : after(1,sec)[op1==50]
    (junction 90) -> four1
    five1 -> three1 : after(1,sec)[op1==25]
    four2 -> five2 : after(1,sec)[op1==25]
    four -> five : after(1,sec)[op1==75]
    four1 -> five1 : after(1,sec)[op1==50]
  (default) -> block_start
  block_start -> Normal2 [order 2] : [data == 0]
  Normal -> Fault [order 1] : [data1 == 1]
  block_start -> Normal [order 1] : [data ==1 ]
  Normal2 -> block_start [order 1] : [data ==1]
  Normal -> block_start [order 2] : [data == 0]
  Fault -> Normal [order 1] : [data1 == 0]
  Fault -> Normal2 [order 2] : [data1 ==0]
  Normal2 -> Fault [order 2] : [data1==1]
  data: data input; data1 input; op1 output =0; warning output

== stateflow chart Automated_features1/MODULES/	POWER_WINDOW/Subsystem4/Rear_right_Subsystem/Chart ==
  state Normal
    state Start
      entry:
      op1 = 25;
    state second
      entry:
      op1 = 100;
    state PrepareToStop
      entry:
      op1 = 75;
    state Go
      % Green light
      entry:
      op1 = 50;
    (default) -> Start
    Start -> (junction 9)
    (junction 9) -> (junction 6) : after(1,sec)
    PrepareToStop -> second : after(1,sec)
    (junction 6) -> Go
    Go -> PrepareToStop : after(1,sec)
  state Fault
    entry:
    op1 =0;
    state BlinkOn
      % Red light
      entry:
      warning = 1;
    (default) -> BlinkOn
  state block_start
    entry:
  state Normal2
    state state5
      entry:
      op1=0
    state Start1
      entry:
    state two
      entry:
      op1 = 0;
    state four3
      entry:
      op1 = 0;
    state three
      entry:
      op1 = 25;
    state three1
      entry:
      op1 = 0;
    state five2
      entry:
      op1=0;
    state five
      entry:
      op1=50;
    state five1
      entry:
      op1=25;
    state four2
      entry:
      op1 = 25;
    state four
      entry:
      op1 = 75;
    state four1
      entry:
      op1 = 50;
    Start1 -> state5 [order 2] : [op1==0]
    (default) -> Start1
    Start1 -> (junction 143) [order 3] : after(1,sec)[op1==25]
    (junction 143) -> four3
    Start1 -> (junction 89) [order 4]
    Start1 -> (junction 103) [order 5]
    Start1 -> (junction 48) [order 1]
    (junction 103) -> (junction 104) : after(1,sec)[op1==50]
    (junction 48) -> (junction 49) : after(1,sec)[op1==100]
    (junction 89) -> (junction 90) : after(1,sec)[op1==75]
    three -> two : after(1,sec)[op1==25]
    (junction 104) -> four2
    (junction 49) -> four
    five -> three : after(1,sec)[op1==50]
    (junction 90) -> four1
    five1 -> three1 : after(1,sec)[op1==25]
    four2 -> five2 : after(1,sec)[op1==25]
    four -> five : after(1,sec)[op1==75]
    four1 -> five1 : after(1,sec)[op1==50]
  (default) -> block_start
  block_start -> Normal2 [order 2] : [data == 0]
  Normal -> Fault [order 1] : [data1 == 1]
  block_start -> Normal [order 1] : [data ==1]
  Normal2 -> block_start [order 1] : [data ==1]
  Normal -> block_start [order 2] : [data ==0]
  Fault -> Normal [order 1] : [data1 == 0]
  Fault -> Normal2 [order 2] : [data1 ==0]
  Normal2 -> Fault [order 2] : [data1==1]
  data: data input; data1 input; op1 output =0; warning output

== stateflow chart Automated_features1/MODULES/	POWER_WINDOW/Subsystem4/driver_control_Subsystem/Chart ==
  state Normal
    state Start
      entry:
      op1 = 25;
    state second
      entry:
      op1 = 100;
    state PrepareToStop
      entry:
      op1 = 75;
    state Go
      % Green light
      entry:
      op1 = 50;
    (default) -> Start
    Start -> (junction 9)
    (junction 9) -> (junction 6) : after(1,sec)
    PrepareToStop -> second : after(1,sec)
    (junction 6) -> Go
    Go -> PrepareToStop : after(1,sec)
  state Fault
    entry:
    op1 =0;
    state BlinkOn
      % Red light
      entry:
      warning = 1;
    (default) -> BlinkOn
  state block_start
    entry:
  state Normal2
    state state5
      entry:
      op1=0
    state Start1
      entry:
      op1=op1;
    state two
      entry:
      op1 = 0;
    state four3
      entry:
      op1 = 0;
    state three
      entry:
      op1 = 25;
    state three1
      entry:
      op1 = 0;
    state five2
      entry:
      op1=0;
    state five
      entry:
      op1=50;
    state five1
      entry:
      op1=25;
    state four2
      entry:
      op1 = 25;
    state four
      entry:
      op1 = 75;
    state four1
      entry:
      op1 = 50;
    Start1 -> state5 [order 4] : [op1==0]
    (default) -> Start1
    Start1 -> (junction 142) [order 2] : after(1,sec)[op1==25]
    Start1 -> (junction 89) [order 3]
    Start1 -> (junction 103) [order 5]
    (junction 142) -> four3
    Start1 -> (junction 48) [order 1]
    (junction 103) -> (junction 104) : after(1,sec)[op1==50]
    (junction 48) -> (junction 49) : after(1,sec)[op1==100]
    (junction 89) -> (junction 90) : after(1,sec)[op1==75]
    three -> two : after(1,sec)[op1==25]
    (junction 104) -> four2
    (junction 49) -> four
    five -> three : after(1,sec)[op1==50]
    (junction 90) -> four1
    five1 -> three1 : after(1,sec)[op1==25]
    four2 -> five2 : after(1,sec)[op1==25]
    four -> five : after(1,sec)[op1==75]
    four1 -> five1 : after(1,sec)[op1==50]
  (default) -> block_start
  block_start -> Normal2 [order 2] : [data == 0]
  Normal -> Fault [order 1] : [data1 == 1]
  block_start -> Normal [order 1] : [data ==1]
  Normal2 -> block_start [order 1] : [data ==1]
  Normal -> block_start [order 2] : [data ==0]
  Fault -> Normal [order 1] : [data1 == 0]
  Fault -> Normal2 [order 2] : [data1 ==0]
  Normal2 -> Fault [order 2] : [data1==1]
  data: data input; data1 input; op1 output =0; warning output

== stateflow chart Automated_features1/MODULES/	POWER_WINDOW/Subsystem4/rear_left_Subsystem/Chart ==
  state Normal
    state Start
      entry:
      op1 = 25;
    state second
      entry:
      op1 = 100;
    state PrepareToStop
      entry:
      op1 = 75;
    state Go
      % Green light
      entry:
      op1 = 50;
    (default) -> Start
    Start -> (junction 9)
    (junction 9) -> (junction 6) : after(1,sec)
    PrepareToStop -> second : after(1,sec)
    (junction 6) -> Go
    Go -> PrepareToStop : after(1,sec)
  state Fault
    entry:
    op1 =0;
    state BlinkOn
      % Red light
      entry:
      warning = 1;
    (default) -> BlinkOn
  state block_start
    entry:
  state Normal2
    state state5
      entry:
      op1=0
    state Start1
      entry:
      op1=op1;
    state two
      entry:
      op1 = 0;
    state four3
      entry:
      op1 = 0;
    state three
      entry:
      op1 = 25;
    state three1
      entry:
      op1 = 0;
    state five2
      entry:
      op1=0;
    state five
      entry:
      op1=50;
    state five1
      entry:
      op1=25;
    state four2
      entry:
      op1 = 25;
    state four
      entry:
      op1 = 75;
    state four1
      entry:
      op1 = 50;
    Start1 -> state5 [order 4] : [op1==0]
    (default) -> Start1
    Start1 -> (junction 142) [order 2] : after(1,sec)[op1==25]
    (junction 142) -> four3
    Start1 -> (junction 89) [order 3]
    Start1 -> (junction 103) [order 5]
    Start1 -> (junction 48) [order 1]
    (junction 103) -> (junction 104) : after(1,sec)[op1==50]
    (junction 48) -> (junction 49) : after(1,sec)[op1==100]
    (junction 89) -> (junction 90) : after(1,sec)[op1==75]
    three -> two : after(1,sec)[op1==25]
    (junction 104) -> four2
    (junction 49) -> four
    five -> three : after(1,sec)[op1==50]
    (junction 90) -> four1
    five1 -> three1 : after(1,sec)[op1==25]
    four2 -> five2 : after(1,sec)[op1==25]
    four -> five : after(1,sec)[op1==75]
    four1 -> five1 : after(1,sec)[op1==50]
  (default) -> block_start
  block_start -> Normal2 [order 2] : [data == 0]
  Normal -> Fault [order 1] : [data1 == 1]
  block_start -> Normal [order 1] : [data ==1]
  Normal2 -> block_start [order 1] : [data ==1]
  Normal -> block_start [order 2] : [data ==0]
  Fault -> Normal [order 1] : [data1 == 0]
  Fault -> Normal2 [order 2] : [data1 ==0]
  Normal2 -> Fault [order 2] : [data1==1]
  data: data input; data1 input; op1 output =0; warning output
